simulink model "mpc_economicEO"  (R2023a)
settings: Solver=ode15s  StartTime=0.0  StopTime=300  MaxStep=5  RelTol=1e-3
values from neighbouring files (symbols this model uses):
  C2H4Avalability = 0.175    [EconomicMPCControlOfEO1.m]
  Tc = 1.1    [EconomicMPCControlOfEO1.m]
  u0 = 0.5    [EconomicMPCControlOfEO1.m]
  x0 = real(fsolve(@(x) oxidationPlantCT(x,[u0;Tc;C2H4Avalability]),rand(1,4),optimopt))    [EconomicMPCControlOfEO1.m]
libraries: mpclib x1
settings Model: Creator=The MathWorks, Inc.  LastModifiedBy=The MathWorks, Inc.
settings SolverCC: AlgebraicLoopSolver=TrustRegion
settings DataIOCC: SaveFormat=Array  SaveOutput=off  SignalLogging=off  DSMLogging=off  SaveTime=off  ReturnWorkspaceOutputs=off
settings OptimizationCC: ReuseModelBlockBuffer=off
settings DebuggingCC: UnconnectedInputMsg=warning  UnconnectedOutputMsg=warning  UnconnectedLineMsg=warning  ArithmeticOperatorsInVariantConditions=warning
settings ModelReferenceCC: EnableRefExpFcnMdlSchedulingChecks=on
settings SFSimCC: SimUseLocalCustomCode=off  CustomCodeUndefinedFunction=UseInterfaceOnly
settings RTWCC: RTWUseLocalCustomCode=off  DLArmComputeVersion=19.05
settings CodeAppCC: StateflowObjectComments=on
settings GRTTargetCC: TargetLangStandard=C89/C90 (ANSI)
settings ConfigComp: CovMetricSettings=dsw  CovSaveCumulativeToWorkspaceVar=on  CovSaveSingleToWorkspaceVar=on  CovExternalEMLEnable=off

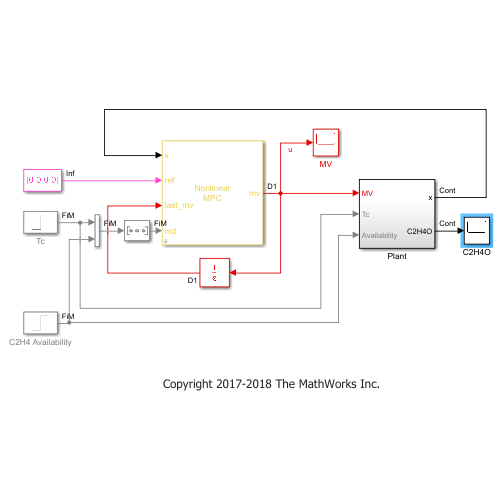
[thumbnail: Simulink's stored preview of the top-level diagram]
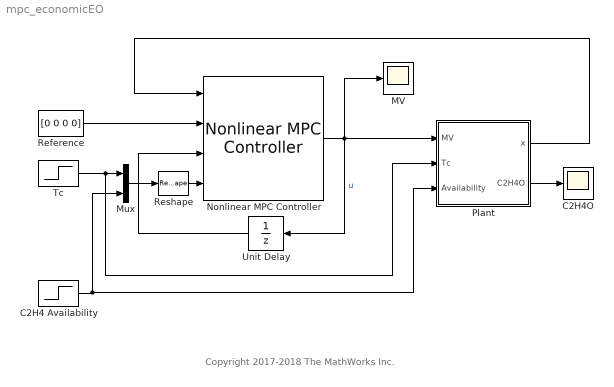
== system mpc_economicEO ==
  note: Copyright 2017-2018 The MathWorks Inc.
  C2H4 Availability : Step  Time=200  Before=C2H4Avalability  After=0.25  SampleTime=0
  C2H4O : Scope
  MV : Scope
  Mux : Mux  Inputs=2
  Nonlinear MPC Controller : mpclib/Nonlinear MPC Controller  SCDEnableBlockLinearizationSpecification=on  nlmpcobj=nlobj  UseObjectTs=on  UseMEX=off  md_enabled=on  mvtarget_enabled=off  param_enabled=off  cost_enabled=off  mvseq_enabled=off  stateseq_enabled=off  ovseq_enabled=off  slack_enabled=off  status_enabled=off  ov_min=off  ov_max=off  mv_min=off  mv_max=off  mvrate_min=off  mvrate_max=off  state_min=off  state_max=off  ov_weight=off  mv_weight=off  mvrate_weight=off  ecr_weight=off  nlp_initialize=off
  Plant : Subsystem
  Reference : Constant  Value=[0 0 0 0]  VectorParams1D=off
  Reshape : Reshape  OutputDimensionality=Row vector (2-D)
  Tc : Step  Time=100  Before=Tc  After=1.15  SampleTime=0
  Unit Delay : UnitDelay  InitialCondition=u0  SampleTime=-1  HasFrameUpgradeWarning=on
  wires:
  Plant/1(x) -> Nonlinear MPC Controller/1
  Tc/1 -> Plant/2(Tc), Mux/1
  Nonlinear MPC Controller/1 -> Unit Delay/1, Plant/1(MV), MV/1  "u"
  Reference/1 -> Nonlinear MPC Controller/2
  Mux/1 -> Reshape/1
  C2H4 Availability/1 -> Mux/2, Plant/3(Availability)
  Plant/2(C2H4O) -> C2H4O/1
  Reshape/1 -> Nonlinear MPC Controller/4
  Unit Delay/1 -> Nonlinear MPC Controller/3

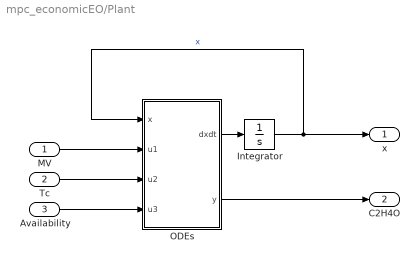
== system mpc_economicEO/Plant ==
  MV : Inport
  Tc : Inport  Port=2
  Availability : Inport  Port=3
  Integrator : Integrator  InitialCondition=x0
  ODEs : MATLAB Function  TreatAsAtomicUnit=on
  x : Outport  VectorParamsAs1DForOutWhenUnconnected=off
  C2H4O : Outport  Port=2  VectorParamsAs1DForOutWhenUnconnected=off
  wires:
  Integrator/1 -> ODEs/1(x), x/1  "x"
  ODEs/1(dxdt) -> Integrator/1
  MV/1 -> ODEs/2(u1)
  Tc/1 -> ODEs/3(u2)
  Availability/1 -> ODEs/4(u3)
  ODEs/2(y) -> C2H4O/1

== matlab function mpc_economicEO/Plant/ODEs ==
  data: dxdt output; x input; u1 input; u2 input; u3 input; y output
function [dxdt, y] = fcn(x, u1, u2, u3)
% Compute time derivatives and outputs for the ethylene oxide reactor
dxdt = oxidationPlantCT(x, [u1;u2;u3]);
y = u3/u1*x(3)*x(4);
